simulink model "btp_VERSION2_final"  (R2020a)
settings: Solver=VariableStepAuto  StartTime=0.0  StopTime=14000  RelTol=1e-3
PreLoadFcn:
  | building_length = 15; % m
  | building_width = 10; % m
  | building_height = 2.5; % m
  | 
  | wall_thickness = 0.2; % m
  | wall_density = 2000; % kg/m^3
  | wall_specific_heat = 840; % J/(kg*K)
  | wall_conductivity = 0.04; % W/(m*K)
  | wall_heat_transfer_coeff_internal = 25; % W/(m^2*K)
  | wall_heat_transfer_coeff_external = 35; % W/(m^2*K)
  | 
  | roof_thickness = 0.2; % m
  | roof_density = 2000; % kg/m^3
  | roof_specific_heat = 840; % J/(kg*K)
  | roof_conductivity = 0.035; % W/(m*K)
  | roof_heat_transfer_coeff_internal = 10; % W/(m^2*K)
  | roof_heat_transfer_coeff_external = 30; % W/(m^2*K)
  | 
  | floor_thickness = 0.1; % m
  | floor_conductivity = 0.15; % W/(m*K)
  | floor_heat_transfer_coeff_internal = 15; % W/(m^2*K)
  | 
  | door_area = 2*0.6; % m^2
  | 
  | duct_area = 0.1^2; % m^2
  | 
  | fan_setting_table = 0 : 4; % 1
  | fan_flow_rate_table = [0 0.08 0.12 0.16 0.2]; % kg/s
  | 
  | initial_temperature = 35; % degC
  | ground_temperature = 25; % degC
  | 
  | flow_reversal_Mach = 1e-5; % 1
InitFcn:
  | zone_volume = building_length * building_width * building_height / 4; % m^3
  | zone_flow_area = 0.7 * building_height * (building_length + building_width) / 4; % m^2
model workspace (MAT data in the model file):
  building_height = 3
  building_length = 4.4
  building_width = 4
  door_area : Simulink.Parameter (value not decoded)
  duct_area = 0.02
  fan_flow_rate_table = [0 0.08 0.12 0.16 0.2]
  fan_setting_table = [0 1 2 3 4]
  floor_conductivity = 0.15
  floor_heat_transfer_coeff_internal = 15
  floor_thickness = 0.1
  flow_reversal_Mach = 1e-05
  ground_temperature = 27
  initial_temperature = 35
  roof_conductivity = 0.04
  roof_density = 2000
  roof_heat_transfer_coeff_external = 30
  roof_heat_transfer_coeff_internal = 10
  roof_specific_heat = 840
  roof_thickness = 0.2
  simlog_ssc_building_ventilation : simscape.logging.Node (value not decoded)
  tout = [0 3.15544362088e-30 8.45959628835e-09 2.5378788865e-08 3.73619145974e-08 4.93450403297e-08 6.73197289282e-08 8.52944175267e-08 1.12256450424e-07 1.39218483322e-07 1.6618051622e-07 1.93142549118e-07 ... (463 elements, 463x1)]
  wall_conductivity = 0.04
  wall_density = 2000
  wall_heat_transfer_coeff_external = 35
  wall_heat_transfer_coeff_internal = 25
  wall_specific_heat = 840
  wall_thickness = 0.2
  zone_flow_area = 9
  zone_volume = 50
undefined symbols (not defined in the file): dbresponses22S1, sigbuilder_block
libraries: fl_lib x53, nesl_utility x27, HVAC_lib x2, simulink x2, fuzblock x1
(part 2 of 2)

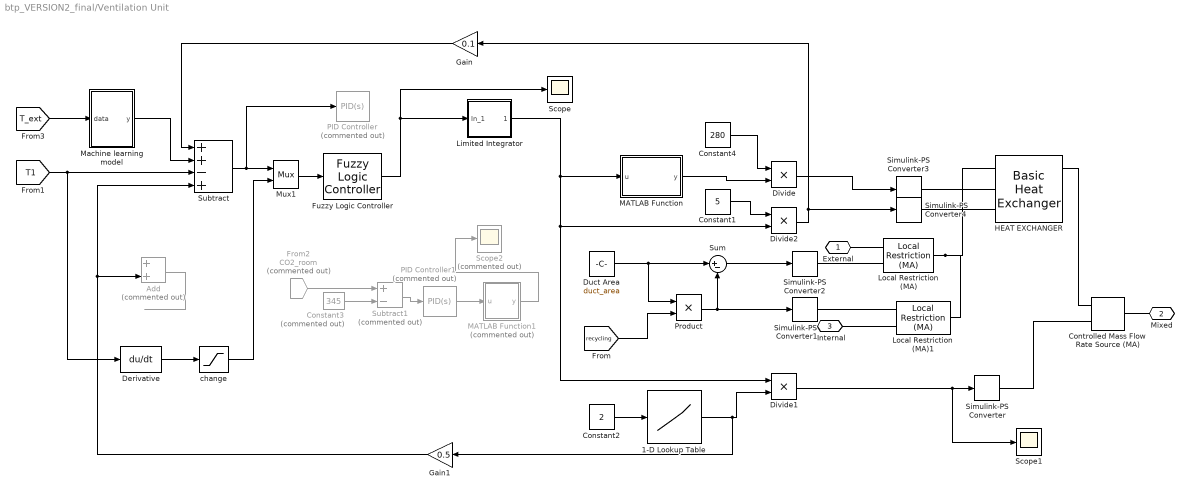
== system btp_VERSION2_final/Ventilation Unit ==
  1-D Lookup Table : Lookup_n-D  NumberOfTableDimensions=1  BreakpointsForDimension1=fan_setting_table  Table=fan_flow_rate_table  ExtrapMethod=Clip  InternalRulePriority=Speed  RndMeth=Simplest  InputSameDT=on
  Add : Sum  Commented=on
  Constant1 : Constant  Value=5
  Constant2 : Constant  Value=2
  Constant3 : Constant  Commented=on  Value=345
  Constant4 : Constant  Value=280
  Controlled Mass Flow Rate Source (MA) : fl_lib/Moist Air/Sources/Controlled Mass Flow Rate Source (MA)  power_spec=foundation.enum.power_spec.isentropic  area_A=duct_area m^2  area_B=duct_area m^2
      settings: SourceProductBaseCode=SS  InternalSimscapePortConfiguration="{\"Bottom\":[],\"Left\":[{\"id\":\"A\",\"label\":\"A\",\"type\":\"foundation.moist_air.moist_air\"},{\"id\":\"M\",\"label\":\"M\",\"type\":\"input\"}],\"Right\":[{\"id\":\"B\",\"label\":\"B\",\"type\":\"foundation.moist_air.moist_air\"}],\"Top\":[]}"
  Derivative : Derivative
  Divide : Product  Inputs=**
  Divide1 : Product  Inputs=**
  Divide2 : Product  Inputs=**
  Duct Area : Constant  Value=duct_area
  From2 : From  Commented=on  GotoTag=CO2_room  TagVisibility=global
  Fuzzy Logic Controller : fuzblock/Fuzzy Logic  Controller  FIS='tipper.fis'  OutputSampleNumber=101  DataType=double  FuzzifiedInputs=off  RuleFiringStrengths=off  RuleOutputs=off  AggregatedOutputs=off  SimulateUsing=Interpreted execution  OutOfRangeInputValueMessage=warning  NoRuleFiredMessage=warning  EmptyOutputFuzzySetMessage=warning
  Gain : Gain  Gain=0.1
  Gain1 : Gain  Gain=0.5
  HEAT EXCHANGER : HVAC_lib/Basic Heat Exchanger  Q_des=6 kW  T1_des=35 degC  mdot1_des=4 kg/s  cp1_des=2 kJ/kg/K  Dp1_des=0.8 kPa  T2_des=300 K  mdot2_des=20 kg/s  cp2_des=10 kJ/kg/K  volume=1e2 m^3  port_area=duct_area m^2  RH_ws=1  time_constant=1e-3 s  p_I_specify=off  p_I_priority=High  p_I=p_env atm  p_I_nominal_specify=off  p_I_nominal_unit=MPa  p_I_nominal_value=1  T_I_specify=on  T_I_priority=High  T_I=initial_temperature degC  T_I_nominal_specify=off  T_I_nominal_unit=K  T_I_nominal_value=1  RH_I_specify=on  RH_I_priority=High  RH_I=0.57  RH_I_nominal_specify=off  RH_I_nominal_unit=1  RH_I_nominal_value=1  x_w_I_specify=off  x_w_I_priority=None  x_w_I=0  x_w_I_nominal_specify=off  x_w_I_nominal_unit=1  x_w_I_nominal_value=1  y_w_I_specify=off  y_w_I_priority=None  y_w_I=0  y_w_I_nominal_specify=off  y_w_I_nominal_unit=1  y_w_I_nominal_value=1  HR_I_specify=off  HR_I_priority=None  HR_I=0  HR_I_nominal_specify=off  HR_I_nominal_unit=1  HR_I_nominal_value=1  x_g_I_specify=off  x_g_I_priority=None  x_g_I=0  x_g_I_nominal_specify=off  x_g_I_nominal_unit=1  x_g_I_nominal_value=1  y_g_I_specify=on  y_g_I_priority=None  y_g_I=0.00045  y_g_I_nominal_specify=off  y_g_I_nominal_unit=1  y_g_I_nominal_value=1
      settings: SourceProductBaseCode=SS  InternalSimscapePortConfiguration="{\"Bottom\":[],\"Left\":[{\"id\":\"A\",\"label\":\"A\",\"type\":\"foundation.moist_air.moist_air\"},{\"id\":\"T2\",\"label\":\"T2\",\"type\":\"input\"},{\"id\":\"M2\",\"label\":\"M2\",\"type\":\"input\"}],\"Right\":[{\"id\":\"B\",\"label\":\"B\",\"type\":\"foundation.moist_air.moist_air\"},{\"id\":\"W\",\"label\":\"W\",\"type\":\"output\"},{\"id\":\"F\",\"label\":\"F\",\"type\":\"output\"}],\"Top\":[]}"
  Limited Integrator : Subsystem  mask(Limited integrator.){lb=0.45, ub=2.95, xi=1}
      mask prompts: lb "Lower bound:"; ub "Upper bound:"; xi "Initial condition"
      mask help: Limited integrator
      mask Help: Implements a limited integrator with \nan expression of the form:\n\nif(x<=lb and u<0) or (x>=ub and u>0)\n\txdot=0\nelse\n\txdot=u.
      mask Display: plot(-1,-0.2,3.5,1.2,[0.05,1,2,2.9],[0,0,1,1]);disp(' 1/s    ')
  Local Restriction (MA) : fl_lib/Moist Air/Elements/Local Restriction (MA)  restriction_type=foundation.enum.restriction_type.variable  restriction_area=0.001 m^2  min_area=1e-10 m^2  max_area=0.99*duct_area m^2  area=duct_area m^2  Cd=0.8  B_lam=0.999
      settings: SourceProductBaseCode=SS
  Local Restriction (MA)1 : fl_lib/Moist Air/Elements/Local Restriction (MA)  restriction_type=foundation.enum.restriction_type.variable  restriction_area=0.001 m^2  min_area=1e-10 m^2  max_area=0.99 * duct_area m^2  area=duct_area m^2  Cd=0.8  B_lam=0.999
      settings: SourceProductBaseCode=SS
  MATLAB Function : MATLAB Function  TreatAsAtomicUnit=on
  MATLAB Function1 : MATLAB Function  Commented=on  TreatAsAtomicUnit=on
  Machine learning model : Subsystem
  Mux1 : Mux  Inputs=2
  PID Controller : simulink/Continuous/PID Controller  Commented=on  Controller=PID  Form=Parallel  TimeDomain=Continuous-time  UseExternalTs=off  SampleTime=-1  IntegratorMethod=Forward Euler  FilterMethod=Forward Euler  ControllerParametersSource=internal  P=4.6  I=0  D=0  UseFilter=on  N=100  TunerSelectOption=Transfer Function Based (PID Tuner App)  InitialConditionSource=internal  InitialConditionForIntegrator=0  InitialConditionForFilter=0  DifferentiatorICPrevScaledInput=0  ExternalReset=none  TrackingMode=off  Kt=1  LimitOutput=on  UpperSaturationLimit=1.25  LowerSaturationLimit=0.75  LinearizeAsGain=on  AntiWindupMode=none  Kb=1  POutMin=[]  POutMax=[]  IOutMin=[]  IOutMax=[]  DOutMin=[]  DOutMax=[]  NOutMin=[]  NOutMax=[]  SumOutMin=[]  SumOutMax=[]  SaturationOutMin=[]  SaturationOutMax=[]  PParamMin=[]  PParamMax=[]  IParamMin=[]  IParamMax=[]  DParamMin=[]  DParamMax=[]  NParamMin=[]  NParamMax=[]  KbParamMin=[]  KbParamMax=[]  KtParamMin=[]  KtParamMax=[]  KbOutMin=[]  KbOutMax=[]  KtOutMin=[]  KtOutMax=[]  IntegratorOutMin=[]  IntegratorOutMax=[]  FilterOutMin=[]  FilterOutMax=[]  SumI1OutMin=[]  SumI1OutMax=[]  SumI2OutMin=[]  SumI2OutMax=[]  SumI3OutMin=[]  SumI3OutMax=[]  SumI4OutMin=[]  SumI4OutMax=[]  SumDOutMin=[]  SumDOutMax=[]  DifferentiatorOutMin=[]  DifferentiatorOutMax=[]  FilterDiffOutCoefMin=[]  FilterDiffOutCoefMax=[]  ReciprocalOutMin=[]  ReciprocalOutMax=[]  SumDenOutMin=[]  SumDenOutMax=[]  SumNumOutMin=[]  SumNumOutMax=[]  DivideOutMin=[]  DivideOutMax=[]  UdiffTsProdOutMin=[]  UdiffTsProdOutMax=[]  NTsProdOutMin=[]  NTsProdOutMax=[]  UintegralTsProdOutMin=[]  UintegralTsProdOutMax=[]  UngainTsProdOutMin=[]  UngainTsProdOutMax=[]  IntegratorContinuousStateAttributes=''  IntegratorStateMustResolveToSignalObject=off  IntegratorRTWStateStorageClass=Auto  FilterContinuousStateAttributes=''  FilterStateMustResolveToSignalObject=off  FilterRTWStateStorageClass=Auto  ParallelPVariant=InternalParameters  IdealPVariant=Disabled  IVariant=InternalParameters  DVariant=InternalParameters  IntegratorVariant=Continuous  SatVariant=Enabled  AWVariant=Passthrough  PCopyVariant=Disabled  TRVariant=Disabled  FdbkBlocksVariant=Forward  IdealPFdbkVariant=Disabled  SatFdbkVariant=Disabled  DerivativeFilterVariant=ContFilter  NVariant=InternalParameters  NCopyVariant=Disabled  FilterICVariant=InternalICsFilter  IntegratorICVariant=InternalICs  ExternalResetVariant=Disabled  TRSumVariant=Passthrough  SumFdbkVariant=Disabled  SumVariant=Sum_PID  TsampFilterVariant=InternalTs  TsampNgainVariant=Passthrough  TsampIntegralVariant=Passthrough
  PID Controller1 : simulink/Continuous/PID Controller  Commented=on  Controller=PID  Form=Parallel  TimeDomain=Continuous-time  UseExternalTs=off  SampleTime=-1  IntegratorMethod=Forward Euler  FilterMethod=Forward Euler  ControllerParametersSource=internal  P=5  I=0.02  D=0  UseFilter=on  N=100  TunerSelectOption=Transfer Function Based (PID Tuner App)  InitialConditionSource=internal  InitialConditionForIntegrator=0  InitialConditionForFilter=0  DifferentiatorICPrevScaledInput=0  ExternalReset=none  TrackingMode=off  Kt=1  LimitOutput=on  UpperSaturationLimit=1.20  LowerSaturationLimit=0.8  LinearizeAsGain=on  AntiWindupMode=none  Kb=1  POutMin=[]  POutMax=[]  IOutMin=[]  IOutMax=[]  DOutMin=[]  DOutMax=[]  NOutMin=[]  NOutMax=[]  SumOutMin=[]  SumOutMax=[]  SaturationOutMin=[]  SaturationOutMax=[]  PParamMin=[]  PParamMax=[]  IParamMin=[]  IParamMax=[]  DParamMin=[]  DParamMax=[]  NParamMin=[]  NParamMax=[]  KbParamMin=[]  KbParamMax=[]  KtParamMin=[]  KtParamMax=[]  KbOutMin=[]  KbOutMax=[]  KtOutMin=[]  KtOutMax=[]  IntegratorOutMin=[]  IntegratorOutMax=[]  FilterOutMin=[]  FilterOutMax=[]  SumI1OutMin=[]  SumI1OutMax=[]  SumI2OutMin=[]  SumI2OutMax=[]  SumI3OutMin=[]  SumI3OutMax=[]  SumI4OutMin=[]  SumI4OutMax=[]  SumDOutMin=[]  SumDOutMax=[]  DifferentiatorOutMin=[]  DifferentiatorOutMax=[]  FilterDiffOutCoefMin=[]  FilterDiffOutCoefMax=[]  ReciprocalOutMin=[]  ReciprocalOutMax=[]  SumDenOutMin=[]  SumDenOutMax=[]  SumNumOutMin=[]  SumNumOutMax=[]  DivideOutMin=[]  DivideOutMax=[]  UdiffTsProdOutMin=[]  UdiffTsProdOutMax=[]  NTsProdOutMin=[]  NTsProdOutMax=[]  UintegralTsProdOutMin=[]  UintegralTsProdOutMax=[]  UngainTsProdOutMin=[]  UngainTsProdOutMax=[]  IntegratorContinuousStateAttributes=''  IntegratorStateMustResolveToSignalObject=off  IntegratorRTWStateStorageClass=Auto  FilterContinuousStateAttributes=''  FilterStateMustResolveToSignalObject=off  FilterRTWStateStorageClass=Auto  ParallelPVariant=InternalParameters  IdealPVariant=Disabled  IVariant=InternalParameters  DVariant=InternalParameters  IntegratorVariant=Continuous  SatVariant=Enabled  AWVariant=Passthrough  PCopyVariant=Disabled  TRVariant=Disabled  FdbkBlocksVariant=Forward  IdealPFdbkVariant=Disabled  SatFdbkVariant=Disabled  DerivativeFilterVariant=ContFilter  NVariant=InternalParameters  NCopyVariant=Disabled  FilterICVariant=InternalICsFilter  IntegratorICVariant=InternalICs  ExternalResetVariant=Disabled  TRSumVariant=Passthrough  SumFdbkVariant=Disabled  SumVariant=Sum_PID  TsampFilterVariant=InternalTs  TsampNgainVariant=Passthrough  TsampIntegralVariant=Passthrough
  Product : Product
  Scope : Scope
  Scope1 : Scope
  Scope2 : Scope  Commented=on
  Simulink-PS Converter : nesl_utility/Simulink-PS Converter  PhysicalDomain=network_engine_domain  SubClassName=ps_input  LeftPortType=input  RightPortType=output  PseudoPeriodic=off  Frequencies=[]  NoiseDistribution=none  NoiseParameters=[]  Unit=kg/s  AffineConversion=off  FilteringAndDerivatives=provide  SimscapeFilterOrder=1  InputFilterTimeConstant=0.001  UdotUserProvided=0
  Simulink-PS Converter1 : nesl_utility/Simulink-PS Converter  PhysicalDomain=network_engine_domain  SubClassName=ps_input  LeftPortType=input  RightPortType=output  PseudoPeriodic=off  Frequencies=[]  NoiseDistribution=none  NoiseParameters=[]  Unit=m^2  AffineConversion=off  FilteringAndDerivatives=provide  SimscapeFilterOrder=1  InputFilterTimeConstant=0.001  UdotUserProvided=0
  Simulink-PS Converter2 : nesl_utility/Simulink-PS Converter  PhysicalDomain=network_engine_domain  SubClassName=ps_input  LeftPortType=input  RightPortType=output  PseudoPeriodic=off  Frequencies=[]  NoiseDistribution=none  NoiseParameters=[]  Unit=m^2  AffineConversion=off  FilteringAndDerivatives=provide  SimscapeFilterOrder=1  InputFilterTimeConstant=0.001  UdotUserProvided=0
  Simulink-PS Converter3 : nesl_utility/Simulink-PS Converter  PhysicalDomain=network_engine_domain  SubClassName=ps_input  LeftPortType=input  RightPortType=output  PseudoPeriodic=off  Frequencies=[]  NoiseDistribution=none  NoiseParameters=[]  Unit=K  AffineConversion=on  FilteringAndDerivatives=provide  SimscapeFilterOrder=1  InputFilterTimeConstant=0.001  UdotUserProvided=0
  Simulink-PS Converter4 : nesl_utility/Simulink-PS Converter  PhysicalDomain=network_engine_domain  SubClassName=ps_input  LeftPortType=input  RightPortType=output  PseudoPeriodic=off  Frequencies=[]  NoiseDistribution=none  NoiseParameters=[]  Unit=kg/s  AffineConversion=on  FilteringAndDerivatives=provide  SimscapeFilterOrder=1  InputFilterTimeConstant=0.001  UdotUserProvided=0
  Subtract : Sum  Inputs=++-+
  Subtract1 : Sum  Commented=on  Inputs=+-
  Sum : Sum  Inputs=|+-
  change : Saturate  UpperLimit=2  LowerLimit=-2
  External : PMIOPort  Side=Left
  Mixed : PMIOPort  Port=2  Side=Right
  Internal : PMIOPort  Port=3  Side=Left
  wires:
  Product/1 -> Sum/2, Simulink-PS Converter1/1
  Sum/1 -> Simulink-PS Converter2/1
  Duct Area/1 -> Product/1, Sum/1
  Constant4/1 -> Divide/1
  [T1] -> Derivative/1, Subtract/3
  Subtract/1 -> PID Controller/1, Mux1/1
  Divide2/1 -> Gain/1, Simulink-PS Converter4/1
  Divide/1 -> Simulink-PS Converter3/1
  Divide1/1 -> Simulink-PS Converter/1, Scope1/1
  Constant2/1 -> 1-D Lookup Table/1
  Constant3/1 -> Subtract1/2
  From2/1 -> Subtract1/1
  Subtract1/1 -> PID Controller1/1
  PID Controller1/1 -> MATLAB Function1/1(u)
  MATLAB Function1/1(y) -> Scope2/1
  [recycling] -> Product/2
  Gain/1 -> Subtract/1
  1-D Lookup Table/1 -> Gain1/1, Divide1/2
  Gain1/1 -> Add/2, Subtract/4
  Derivative/1 -> change/1
  change/1 -> Mux1/2
  Mux1/1 -> Fuzzy Logic Controller/1
  Fuzzy Logic Controller/1 -> Limited Integrator/1(In_1), Scope/1
  Limited Integrator/1(Out_1) -> MATLAB Function/1(u), Divide2/2, Divide1/1
  Constant1/1 -> Divide2/1
  Machine learning model/1(y) -> Subtract/2
  [T_ext] -> Machine learning model/1(data)
  MATLAB Function/1(y) -> Divide/2
  Add/1 -> ?
  connections:
  Simulink-PS Converter/RConn1 -- Controlled Mass Flow Rate Source (MA)/LConn2
  External/RConn1 -- Local Restriction (MA)/LConn1
  Simulink-PS Converter2/RConn1 -- Local Restriction (MA)/LConn2
  Controlled Mass Flow Rate Source (MA)/RConn1 -- Mixed/RConn1
  Simulink-PS Converter1/RConn1 -- Local Restriction (MA)1/LConn2
  Internal/RConn1 -- Local Restriction (MA)1/LConn1
  Local Restriction (MA)/RConn1 -- HEAT EXCHANGER/LConn1 -- Local Restriction (MA)1/RConn1
  Simulink-PS Converter3/RConn1 -- HEAT EXCHANGER/LConn2
  Simulink-PS Converter4/RConn1 -- HEAT EXCHANGER/LConn3
  HEAT EXCHANGER/RConn1 -- Controlled Mass Flow Rate Source (MA)/LConn1

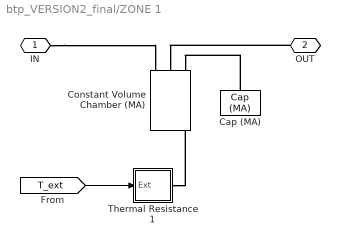
== system btp_VERSION2_final/ZONE 1 ==
  Cap (MA) : fl_lib/Moist Air/Elements/Cap (MA)  p_specify=on  p_priority=None  p=0.101325 MPa  p_nominal_specify=off  p_nominal_unit=MPa  p_nominal_value=1  T_specify=on  T_priority=None  T=initial_temperature K  T_nominal_specify=off  T_nominal_unit=K  T_nominal_value=1  x_w_specify=on  x_w_priority=None  x_w=0.57  x_w_nominal_specify=off  x_w_nominal_unit=1  x_w_nominal_value=1  x_g_specify=on  x_g_priority=None  x_g=0.00045  x_g_nominal_specify=off  x_g_nominal_unit=1  x_g_nominal_value=1
      settings: SourceProductBaseCode=SS  InternalSimscapePortConfiguration="{\"Bottom\":[],\"Left\":[{\"id\":\"A\",\"label\":\"\",\"type\":\"foundation.moist_air.moist_air\"}],\"Right\":[],\"Top\":[]}"
  Constant Volume Chamber (MA) : fl_lib/Moist Air/Elements/Constant Volume Chamber (MA)  volume=zone_volume/2 m^3  num_ports=foundation.enum.num_ports.three  area_A=duct_area m^2  area_B=zone_flow_area m^2  area_C=zone_flow_area m^2  area_D=0.01 m^2  RH_ws=1  time_constant=1e-3 s  moisture_trace_gas_source=foundation.enum.moisture_trace_gas_source.none  moisture_source_spec=foundation.enum.moisture_source_spec.vapor  moisture_mass_flow=0 kg/s  moisture_temperature_spec=foundation.enum.temperature_spec.atmospheric  moisture_temperature=293.15 K  trace_gas_mass_flow=0 kg/s  trace_gas_temperature_spec=foundation.enum.temperature_spec.atmospheric  trace_gas_temperature=293.15 K  p_I_specify=on  p_I_priority=High  p_I=0.101325 MPa  p_I_nominal_specify=off  p_I_nominal_unit=MPa  p_I_nominal_value=1  T_I_specify=on  T_I_priority=None  T_I=initial_temperature K  T_I_nominal_specify=off  T_I_nominal_unit=K  T_I_nominal_value=1  RH_I_specify=on  RH_I_priority=None  RH_I=0.57  RH_I_nominal_specify=off  RH_I_nominal_unit=1  RH_I_nominal_value=1  x_w_I_specify=off  x_w_I_priority=None  x_w_I=0  x_w_I_nominal_specify=off  x_w_I_nominal_unit=1  x_w_I_nominal_value=1  y_w_I_specify=off  y_w_I_priority=None  y_w_I=0  y_w_I_nominal_specify=off  y_w_I_nominal_unit=1  y_w_I_nominal_value=1  HR_I_specify=off  HR_I_priority=None  HR_I=0  HR_I_nominal_specify=off  HR_I_nominal_unit=1  HR_I_nominal_value=1  x_g_I_specify=off  x_g_I_priority=Low  x_g_I=0  x_g_I_nominal_specify=off  x_g_I_nominal_unit=1  x_g_I_nominal_value=1  y_g_I_specify=on  y_g_I_priority=None  y_g_I=0.00045  y_g_I_nominal_specify=off  y_g_I_nominal_unit=1  y_g_I_nominal_value=1
      settings: SourceProductBaseCode=SS  InternalSimscapePortConfiguration="{\"Bottom\":[],\"Left\":[{\"id\":\"A\",\"label\":\"A\",\"type\":\"foundation.moist_air.moist_air\"},{\"id\":\"B\",\"label\":\"B\",\"type\":\"foundation.moist_air.moist_air\"},{\"id\":\"C\",\"label\":\"C\",\"type\":\"foundation.moist_air.moist_air\"}],\"Right\":[{\"id\":\"W\",\"label\":\"W\",\"type\":\"output\"},{\"id\":\"F\",\"label\":\"F\",\"type\":\"output\"},{\"id\":\"H\",\"label\":\"H\",\"type\":\"foundation.thermal.thermal\"}],\"Top\":[]}"
  Thermal Resistance 1 : Subsystem  Tag=PublishSubsystem  mask(Zone Thermal Resistance){zone_length=building_length / 2, zone_width=building_width / 2, zone_height=building_height / 2, wall_thickness=wall_thickness, wall_density=wall_density, wall_specific_heat=wall_specific_heat, wall_conductivity=wall_conductivity, wall_heat_transfer_coeff_internal=wall_heat_transfer_coeff_internal, wall_heat_transfer_coeff_external=wall_heat_transfer_coeff_external, wall_initial_temperature=initial_temperature, roof_thickness=roof_thickness, roof_density=roof_density, roof_specific_heat=roof_specific_heat, roof_conductivity=roof_conductivity, roof_heat_transfer_coeff_internal=roof_heat_transfer_coeff_internal, roof_heat_transfer_coeff_external=roof_heat_transfer_coeff_external, roof_initial_temperature=initial_temperature, floor_thickness=floor_thickness, floor_conductivity=floor_conductivity, floor_heat_transfer_coeff_internal=floor_heat_transfer_coeff_internal, ground_temperature=ground_temperature}
      mask prompts: zone_length "Zone length (m)"; zone_width "Zone width (m)"; zone_height "Zone height (m)"; wall_thickness "Thickness (m)"; wall_density "Density (kg/m^3)"; wall_specific_heat "Specific heat (J/(kg*K))"; wall_conductivity "Thermal conductivity (W/(m*K))"; wall_heat_transfer_coeff_internal "Internal heat transfer coefficient (W/(m^2*K))"; wall_heat_transfer_coeff_external "External heat transfer coefficient (W/(m^2*K))"; wall_initial_temperature "Initial temperature (degC)"; roof_thickness "Thickness (m)"; roof_density "Density (kg/m^3)"; roof_specific_heat "Specific heat (J/(kg*K))"; roof_conductivity "Thermal conductivity (W/(m*K))"; roof_heat_transfer_coeff_internal "Internal heat transfer coefficient (W/(m^2*K))"; roof_heat_transfer_coeff_external "External heat transfer coefficient (W/(m^2*K))"; roof_initial_temperature "Initial temperature (degC)"; floor_thickness "Thickness (m)"; floor_conductivity "Thermal conductivity (W/(m*K))"; floor_heat_transfer_coeff_internal "Internal heat transfer coefficient (W/(m^2*K))"; ground_temperature "Ground temperature (degC)"
      mask help: This subsystem models the thermal resistances of the wall and of the roof between the zone and the external environment. It also models the thermal resistance of the floor between the zone and the ground.
      mask init:
      | wall_area = zone_height * (zone_length + zone_width);
      | roof_area = zone_length * zone_width;
      | floor_area = zone_length * zone_width;
      mask DialogControl TabGeometry Prompt: Geometry
      mask DialogControl TabWall Prompt: Wall
      mask DialogControl TabRoof Prompt: Roof
      mask DialogControl TabFloor Prompt: Floor
  IN : PMIOPort  Side=Left
  OUT : PMIOPort  Port=2  Side=Right
  wires:
  [T_ext] -> Thermal Resistance 1/1(Ext)
  connections:
  OUT/RConn1 -- Constant Volume Chamber (MA)/LConn2
  Cap (MA)/LConn1 -- Constant Volume Chamber (MA)/LConn3
  Thermal Resistance 1/RConn1 -- Constant Volume Chamber (MA)/RConn3
  IN/RConn1 -- Constant Volume Chamber (MA)/LConn1

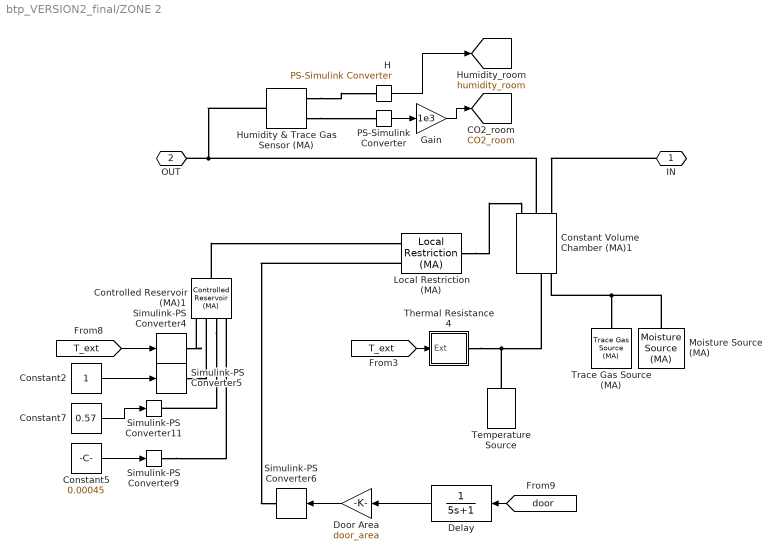
== system btp_VERSION2_final/ZONE 2 ==
  Constant Volume Chamber (MA)1 : fl_lib/Moist Air/Elements/Constant Volume Chamber (MA)  volume=zone_volume/2 m^3  num_ports=foundation.enum.num_ports.three  area_A=duct_area m^2  area_B=zone_flow_area m^2  area_C=zone_flow_area m^2  area_D=0.01 m^2  RH_ws=1  time_constant=1e-3 s  moisture_trace_gas_source=foundation.enum.moisture_trace_gas_source.controlled  moisture_source_spec=foundation.enum.moisture_source_spec.vapor  moisture_mass_flow=0 kg/s  moisture_temperature_spec=foundation.enum.temperature_spec.atmospheric  moisture_temperature=293.15 K  trace_gas_mass_flow=0 kg/s  trace_gas_temperature_spec=foundation.enum.temperature_spec.atmospheric  trace_gas_temperature=293.15 K  p_I_specify=on  p_I_priority=High  p_I=0.101325 MPa  p_I_nominal_specify=off  p_I_nominal_unit=MPa  p_I_nominal_value=1  T_I_specify=on  T_I_priority=High  T_I=initial_temperature K  T_I_nominal_specify=off  T_I_nominal_unit=K  T_I_nominal_value=1  RH_I_specify=on  RH_I_priority=None  RH_I=0.57  RH_I_nominal_specify=off  RH_I_nominal_unit=1  RH_I_nominal_value=1  x_w_I_specify=off  x_w_I_priority=None  x_w_I=0  x_w_I_nominal_specify=off  x_w_I_nominal_unit=1  x_w_I_nominal_value=1  y_w_I_specify=off  y_w_I_priority=None  y_w_I=0  y_w_I_nominal_specify=off  y_w_I_nominal_unit=1  y_w_I_nominal_value=1  HR_I_specify=off  HR_I_priority=None  HR_I=0  HR_I_nominal_specify=off  HR_I_nominal_unit=1  HR_I_nominal_value=1  x_g_I_specify=off  x_g_I_priority=None  x_g_I=0  x_g_I_nominal_specify=off  x_g_I_nominal_unit=1  x_g_I_nominal_value=1  y_g_I_specify=on  y_g_I_priority=None  y_g_I=0.00045  y_g_I_nominal_specify=off  y_g_I_nominal_unit=1  y_g_I_nominal_value=1
      settings: SourceProductBaseCode=SS  InternalSimscapePortConfiguration="{\"Bottom\":[],\"Left\":[{\"id\":\"A\",\"label\":\"A\",\"type\":\"foundation.moist_air.moist_air\"},{\"id\":\"B\",\"label\":\"B\",\"type\":\"foundation.moist_air.moist_air\"},{\"id\":\"C\",\"label\":\"C\",\"type\":\"foundation.moist_air.moist_air\"}],\"Right\":[{\"id\":\"W\",\"label\":\"W\",\"type\":\"output\"},{\"id\":\"F\",\"label\":\"F\",\"type\":\"output\"},{\"id\":\"H\",\"label\":\"H\",\"type\":\"foundation.thermal.thermal\"},{\"id\":\"S\",\"label\":\"S\",\"type\":\"foundation.moist_air.moist_air_source\"}],\"Top\":[]}"
  Constant2 : Constant
  Constant5 : Constant  Value=0.00045
  Constant7 : Constant  Value=0.57
  Controlled Reservoir (MA)1 : fl_lib/Moist Air/Elements/Controlled Reservoir (MA)  moisture_spec=foundation.enum.moisture_spec.relative_humidity  trace_gas_spec=foundation.enum.trace_gas_spec.mole_fraction  RH_ws=1  area_A=duct_area m^2  input_error_spec=foundation.enum.input_range_error.warn
      settings: SourceProductBaseCode=SS  InternalSimscapePortConfiguration="{\"Bottom\":[],\"Left\":[{\"id\":\"A\",\"label\":\"A\",\"type\":\"foundation.moist_air.moist_air\"}],\"Right\":[{\"id\":\"T\",\"label\":\"T\",\"type\":\"input\"},{\"id\":\"P\",\"label\":\"P\",\"type\":\"input\"},{\"id\":\"W\",\"label\":\"W\",\"type\":\"input\"},{\"id\":\"G\",\"label\":\"G\",\"type\":\"input\"}],\"Top\":[]}"
  Delay : TransferFcn  Denominator=[5 1]
  Door Area : Gain  Gain=door_area
  Gain : Gain  Gain=1e3
  H : nesl_utility/PS-Simulink Converter  PhysicalDomain=network_engine_domain  SubClassName=ps_output  LeftPortType=input  RightPortType=output  PseudoPeriodic=off  Frequencies=[]  Unit=1  AffineConversion=off
  Humidity & Trace Gas Sensor (MA) : fl_lib/Moist Air/Sensors/Humidity & Trace Gas Sensor (MA)  moisture_spec=foundation.enum.moisture_spec.relative_humidity  trace_gas_spec=foundation.enum.trace_gas_spec.mole_fraction
      settings: SourceProductBaseCode=SS  InternalSimscapePortConfiguration="{\"Bottom\":[],\"Left\":[{\"id\":\"A\",\"label\":\"A\",\"type\":\"foundation.moist_air.moist_air\"}],\"Right\":[{\"id\":\"W\",\"label\":\"W\",\"type\":\"output\"},{\"id\":\"G\",\"label\":\"G\",\"type\":\"output\"}],\"Top\":[]}"
  Local Restriction (MA) : fl_lib/Moist Air/Elements/Local Restriction (MA)  restriction_type=foundation.enum.restriction_type.variable  restriction_area=0.5 * duct_area m^2  min_area=1e-7 m^2  max_area=0.9*door_area m^2  area=door_area m^2  Cd=0.8  B_lam=0.999
      settings: SourceProductBaseCode=SS
  Moisture Source (MA) : fl_lib/Moist Air/Sources/Moisture & Trace Gas Sources/Moisture Source (MA)  moisture_source_spec=foundation.enum.moisture_source_spec.vapor  moisture_mass_flow=0.015 kg/s  temperature_spec=foundation.enum.temperature_spec.specified  moisture_temperature=303 K
      settings: SourceProductBaseCode=SS  InternalSimscapePortConfiguration="{\"Bottom\":[],\"Left\":[{\"id\":\"S\",\"label\":\"S\",\"type\":\"foundation.moist_air.moist_air_source\"}],\"Right\":[],\"Top\":[]}"
  PS-Simulink Converter : nesl_utility/PS-Simulink Converter  PhysicalDomain=network_engine_domain  SubClassName=ps_output  LeftPortType=input  RightPortType=output  PseudoPeriodic=off  Frequencies=[]  Unit=1  AffineConversion=off
  Simulink-PS Converter11 : nesl_utility/Simulink-PS Converter  PhysicalDomain=network_engine_domain  SubClassName=ps_input  LeftPortType=input  RightPortType=output  PseudoPeriodic=off  Frequencies=[]  NoiseDistribution=none  NoiseParameters=[]  Unit=1  AffineConversion=off  FilteringAndDerivatives=provide  SimscapeFilterOrder=1  InputFilterTimeConstant=0.001  UdotUserProvided=0
  Simulink-PS Converter4 : nesl_utility/Simulink-PS Converter  PhysicalDomain=network_engine_domain  SubClassName=ps_input  LeftPortType=input  RightPortType=output  PseudoPeriodic=off  Frequencies=[]  NoiseDistribution=none  NoiseParameters=[]  Unit=degC  AffineConversion=on  FilteringAndDerivatives=provide  SimscapeFilterOrder=1  InputFilterTimeConstant=0.001  UdotUserProvided=0
  Simulink-PS Converter5 : nesl_utility/Simulink-PS Converter  PhysicalDomain=network_engine_domain  SubClassName=ps_input  LeftPortType=input  RightPortType=output  PseudoPeriodic=off  Frequencies=[]  NoiseDistribution=none  NoiseParameters=[]  Unit=atm  AffineConversion=off  FilteringAndDerivatives=provide  SimscapeFilterOrder=1  InputFilterTimeConstant=0.001  UdotUserProvided=0
  Simulink-PS Converter6 : nesl_utility/Simulink-PS Converter  PhysicalDomain=network_engine_domain  SubClassName=ps_input  LeftPortType=input  RightPortType=output  PseudoPeriodic=off  Frequencies=[]  NoiseDistribution=none  NoiseParameters=[]  Unit=m^2  AffineConversion=off  FilteringAndDerivatives=provide  SimscapeFilterOrder=1  InputFilterTimeConstant=0.001  UdotUserProvided=0
  Simulink-PS Converter9 : nesl_utility/Simulink-PS Converter  PhysicalDomain=network_engine_domain  SubClassName=ps_input  LeftPortType=input  RightPortType=output  PseudoPeriodic=off  Frequencies=[]  NoiseDistribution=none  NoiseParameters=[]  Unit=1  AffineConversion=off  FilteringAndDerivatives=provide  SimscapeFilterOrder=1  InputFilterTimeConstant=0.001  UdotUserProvided=0
  Temperature Source : fl_lib/Thermal/Thermal Sources/Temperature Source  temperature=303 K
  Thermal Resistance 4 : Subsystem  mask(Zone Thermal Resistance){zone_length=building_length / 2, zone_width=building_width / 2, zone_height=building_height / 2, wall_thickness=wall_thickness, wall_density=wall_density, wall_specific_heat=wall_specific_heat, wall_conductivity=wall_conductivity, wall_heat_transfer_coeff_internal=wall_heat_transfer_coeff_internal, wall_heat_transfer_coeff_external=wall_heat_transfer_coeff_external, wall_initial_temperature=initial_temperature, roof_thickness=roof_thickness, roof_density=roof_density, roof_specific_heat=roof_specific_heat, roof_conductivity=roof_conductivity, roof_heat_transfer_coeff_internal=roof_heat_transfer_coeff_internal, roof_heat_transfer_coeff_external=roof_heat_transfer_coeff_external, roof_initial_temperature=initial_temperature, floor_thickness=floor_thickness, floor_conductivity=floor_conductivity, floor_heat_transfer_coeff_internal=floor_heat_transfer_coeff_internal, ground_temperature=ground_temperature}
      mask prompts: zone_length "Zone length (m)"; zone_width "Zone width (m)"; zone_height "Zone height (m)"; wall_thickness "Thickness (m)"; wall_density "Density (kg/m^3)"; wall_specific_heat "Specific heat (J/(kg*K))"; wall_conductivity "Thermal conductivity (W/(m*K))"; wall_heat_transfer_coeff_internal "Internal heat transfer coefficient (W/(m^2*K))"; wall_heat_transfer_coeff_external "External heat transfer coefficient (W/(m^2*K))"; wall_initial_temperature "Initial temperature (degC)"; roof_thickness "Thickness (m)"; roof_density "Density (kg/m^3)"; roof_specific_heat "Specific heat (J/(kg*K))"; roof_conductivity "Thermal conductivity (W/(m*K))"; roof_heat_transfer_coeff_internal "Internal heat transfer coefficient (W/(m^2*K))"; roof_heat_transfer_coeff_external "External heat transfer coefficient (W/(m^2*K))"; roof_initial_temperature "Initial temperature (degC)"; floor_thickness "Thickness (m)"; floor_conductivity "Thermal conductivity (W/(m*K))"; floor_heat_transfer_coeff_internal "Internal heat transfer coefficient (W/(m^2*K))"; ground_temperature "Ground temperature (degC)"
      mask help: This subsystem models the thermal resistances of the wall and of the roof between the zone and the external environment. It also models the thermal resistance of the floor between the zone and the ground.
      mask init:
      | wall_area = zone_height * (zone_length + zone_width);
      | roof_area = zone_length * zone_width;
      | floor_area = zone_length * zone_width;
      mask DialogControl TabGeometry Prompt: Geometry
      mask DialogControl TabWall Prompt: Wall
      mask DialogControl TabRoof Prompt: Roof
      mask DialogControl TabFloor Prompt: Floor
  Trace Gas Source (MA) : fl_lib/Moist Air/Sources/Moisture & Trace Gas Sources/Trace Gas Source (MA)  trace_gas_mass_flow=0.04 kg/s  temperature_spec=foundation.enum.temperature_spec.specified  trace_gas_temperature=303 K
      settings: SourceProductBaseCode=SS  InternalSimscapePortConfiguration="{\"Bottom\":[],\"Left\":[{\"id\":\"S\",\"label\":\"S\",\"type\":\"foundation.moist_air.moist_air_source\"}],\"Right\":[],\"Top\":[]}"
  IN : PMIOPort  Side=Right
  OUT : PMIOPort  Port=2  Side=Left
  tag scope: CO2_room=global, humidity_room=global
  wires:
  Constant2/1 -> Simulink-PS Converter5/1
  Delay/1 -> Door Area/1
  Constant5/1 -> Simulink-PS Converter9/1
  [T_ext] -> Thermal Resistance 4/1(Ext)
  Constant7/1 -> Simulink-PS Converter11/1
  PS-Simulink Converter/1 -> Gain/1
  H/1 -> [humidity_room]
  Door Area/1 -> Simulink-PS Converter6/1
  [T_ext] -> Simulink-PS Converter4/1
  [door] -> Delay/1
  Gain/1 -> [CO2_room]
  connections:
  Controlled Reservoir (MA)1/LConn1 -- Local Restriction (MA)/LConn1
  Humidity & Trace Gas Sensor (MA)/RConn1 -- H/LConn1
  Controlled Reservoir (MA)1/RConn3 -- Simulink-PS Converter11/RConn1
  Simulink-PS Converter9/RConn1 -- Controlled Reservoir (MA)1/RConn4
  Thermal Resistance 4/RConn1 -- Temperature Source/LConn1 -- Constant Volume Chamber (MA)1/RConn3
  Humidity & Trace Gas Sensor (MA)/LConn1 -- Constant Volume Chamber (MA)1/LConn2 -- OUT/RConn1
  Local Restriction (MA)/LConn2 -- Simulink-PS Converter6/RConn1
  Local Restriction (MA)/RConn1 -- Constant Volume Chamber (MA)1/LConn1
  Moisture Source (MA)/LConn1 -- Constant Volume Chamber (MA)1/RConn4 -- Trace Gas Source (MA)/LConn1
  Humidity & Trace Gas Sensor (MA)/RConn2 -- PS-Simulink Converter/LConn1
  Simulink-PS Converter5/RConn1 -- Controlled Reservoir (MA)1/RConn2
  Simulink-PS Converter4/RConn1 -- Controlled Reservoir (MA)1/RConn1
  IN/RConn1 -- Constant Volume Chamber (MA)1/LConn3

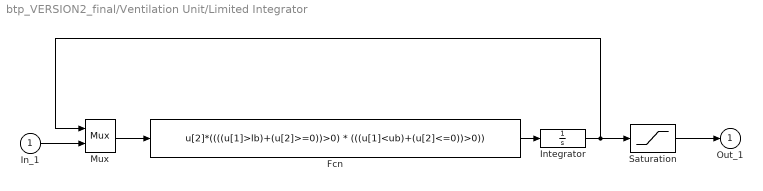
== system btp_VERSION2_final/Ventilation Unit/Limited Integrator ==
  In_1 : Inport
  Fcn : Fcn  Expr=u[2]*((((u[1]>lb)+(u[2]>=0))>0) * (((u[1]<ub)+(u[2]<=0))>0))
  Integrator : Integrator  InitialCondition=xi
  Mux : Mux  Inputs=2
  Saturation : Saturate  UpperLimit=ub  LowerLimit=lb
  Out_1 : Outport  InitialOutput=0  VectorParamsAs1DForOutWhenUnconnected=off
  wires:
  Integrator/1 -> Saturation/1, Mux/1
  Fcn/1 -> Integrator/1
  Mux/1 -> Fcn/1
  In_1/1 -> Mux/2
  Saturation/1 -> Out_1/1

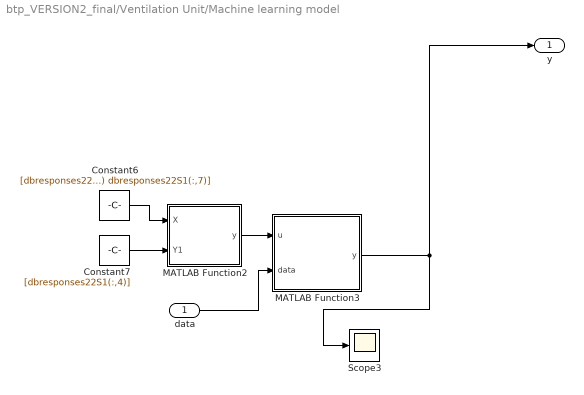
== system btp_VERSION2_final/Ventilation Unit/Machine learning model ==
  data : Inport
  Constant6 : Constant  Value=[dbresponses22S1(:,1) dbresponses22S1(:,2) dbresponses22S1(:,5) dbresponses22S1(:,6) dbresponses22S1(:,7)]
  Constant7 : Constant  Value=[dbresponses22S1(:,4)]
  MATLAB Function2 : MATLAB Function  TreatAsAtomicUnit=on
  MATLAB Function3 : MATLAB Function  TreatAsAtomicUnit=on
  Scope3 : Scope
  y : Outport
  wires:
  MATLAB Function3/1(y) -> y/1, Scope3/1
  MATLAB Function2/1(y) -> MATLAB Function3/1(u)
  Constant6/1 -> MATLAB Function2/1(X)
  data/1 -> MATLAB Function3/2(data)
  Constant7/1 -> MATLAB Function2/2(Y1)

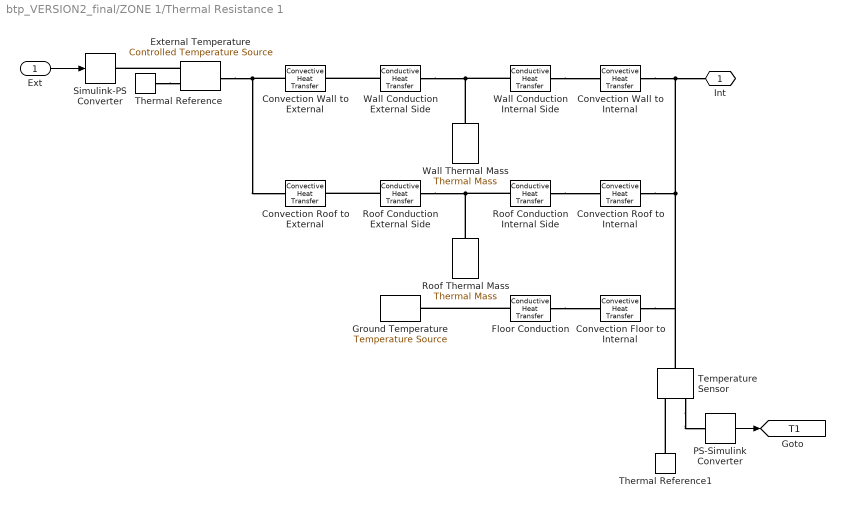
== system btp_VERSION2_final/ZONE 1/Thermal Resistance 1 ==
  Ext : Inport
  Convection Floor to Internal : fl_lib/Thermal/Thermal Elements/Convective Heat Transfer  area=floor_area m^2  heat_tr_coeff=floor_heat_transfer_coeff_internal W/(m^2 * K)  T_specify=off  T_priority=None  T=0 K  T_nominal_specify=off  T_nominal_unit=K  T_nominal_value=1  Q_specify=off  Q_priority=None  Q=0 W  Q_nominal_specify=off  Q_nominal_unit=W  Q_nominal_value=1
  Convection Roof to External : fl_lib/Thermal/Thermal Elements/Convective Heat Transfer  area=roof_area m^2  heat_tr_coeff=roof_heat_transfer_coeff_external W/(m^2 * K)  T_specify=off  T_priority=None  T=0 K  T_nominal_specify=off  T_nominal_unit=K  T_nominal_value=1  Q_specify=off  Q_priority=None  Q=0 W  Q_nominal_specify=off  Q_nominal_unit=W  Q_nominal_value=1
  Convection Roof to Internal : fl_lib/Thermal/Thermal Elements/Convective Heat Transfer  area=roof_area m^2  heat_tr_coeff=roof_heat_transfer_coeff_internal W/(m^2 * K)  T_specify=off  T_priority=None  T=0 K  T_nominal_specify=off  T_nominal_unit=K  T_nominal_value=1  Q_specify=off  Q_priority=None  Q=0 W  Q_nominal_specify=off  Q_nominal_unit=W  Q_nominal_value=1
  Convection Wall to External : fl_lib/Thermal/Thermal Elements/Convective Heat Transfer  area=wall_area m^2  heat_tr_coeff=wall_heat_transfer_coeff_external W/(m^2 * K)  T_specify=off  T_priority=None  T=0 K  T_nominal_specify=off  T_nominal_unit=K  T_nominal_value=1  Q_specify=off  Q_priority=None  Q=0 W  Q_nominal_specify=off  Q_nominal_unit=W  Q_nominal_value=1
  Convection Wall to Internal : fl_lib/Thermal/Thermal Elements/Convective Heat Transfer  area=wall_area m^2  heat_tr_coeff=wall_heat_transfer_coeff_internal W/(m^2 * K)  T_specify=off  T_priority=None  T=0 K  T_nominal_specify=off  T_nominal_unit=K  T_nominal_value=1  Q_specify=off  Q_priority=None  Q=0 W  Q_nominal_specify=off  Q_nominal_unit=W  Q_nominal_value=1
  External Temperature : fl_lib/Thermal/Thermal Sources/Controlled Temperature Source
  Floor Conduction : fl_lib/Thermal/Thermal Elements/Conductive Heat Transfer  area=floor_area m^2  thickness=floor_thickness m  th_cond=floor_conductivity W/(m*K)  T_specify=off  T_priority=None  T=0 K  T_nominal_specify=off  T_nominal_unit=K  T_nominal_value=1  Q_specify=off  Q_priority=None  Q=0 W  Q_nominal_specify=off  Q_nominal_unit=W  Q_nominal_value=1
  Ground Temperature : fl_lib/Thermal/Thermal Sources/Temperature Source  temperature=ground_temperature degC
  PS-Simulink Converter : nesl_utility/PS-Simulink Converter  PhysicalDomain=network_engine_domain  SubClassName=ps_output  LeftPortType=input  RightPortType=output  PseudoPeriodic=off  Frequencies=[]  Unit=degC  AffineConversion=on
  Roof Conduction External Side : fl_lib/Thermal/Thermal Elements/Conductive Heat Transfer  area=roof_area m^2  thickness=roof_thickness / 2 m  th_cond=roof_conductivity W/(m*K)  T_specify=off  T_priority=None  T=0 K  T_nominal_specify=off  T_nominal_unit=K  T_nominal_value=1  Q_specify=off  Q_priority=None  Q=0 W  Q_nominal_specify=off  Q_nominal_unit=W  Q_nominal_value=1
  Roof Conduction Internal Side : fl_lib/Thermal/Thermal Elements/Conductive Heat Transfer  area=roof_area m^2  thickness=roof_thickness / 2 m  th_cond=roof_conductivity W/(m*K)  T_specify=off  T_priority=None  T=0 K  T_nominal_specify=off  T_nominal_unit=K  T_nominal_value=1  Q_specify=off  Q_priority=None  Q=0 W  Q_nominal_specify=off  Q_nominal_unit=W  Q_nominal_value=1
  Roof Thermal Mass : fl_lib/Thermal/Thermal Elements/Thermal Mass  mass=roof_area * roof_thickness * wall_density kg  sp_heat=roof_specific_heat J/kg/K  T_specify=on  T_priority=High  T=roof_initial_temperature degC  T_nominal_specify=off  T_nominal_unit=K  T_nominal_value=1  Q_specify=off  Q_priority=None  Q=0 W  Q_nominal_specify=off  Q_nominal_unit=W  Q_nominal_value=1
  Simulink-PS Converter : nesl_utility/Simulink-PS Converter  PhysicalDomain=network_engine_domain  SubClassName=ps_input  LeftPortType=input  RightPortType=output  PseudoPeriodic=off  Frequencies=[]  NoiseDistribution=none  NoiseParameters=[]  Unit=degC  AffineConversion=on  FilteringAndDerivatives=provide  SimscapeFilterOrder=1  InputFilterTimeConstant=0.001  UdotUserProvided=0
  Temperature Sensor : fl_lib/Thermal/Thermal Sensors/Temperature Sensor
  Thermal Reference : fl_lib/Thermal/Thermal Elements/Thermal Reference
  Thermal Reference1 : fl_lib/Thermal/Thermal Elements/Thermal Reference
  Wall Conduction External Side : fl_lib/Thermal/Thermal Elements/Conductive Heat Transfer  area=wall_area m^2  thickness=wall_thickness / 2 m  th_cond=wall_conductivity W/(m*K)  T_specify=off  T_priority=None  T=0 K  T_nominal_specify=off  T_nominal_unit=K  T_nominal_value=1  Q_specify=off  Q_priority=None  Q=0 W  Q_nominal_specify=off  Q_nominal_unit=W  Q_nominal_value=1
  Wall Conduction Internal Side : fl_lib/Thermal/Thermal Elements/Conductive Heat Transfer  area=wall_area m^2  thickness=wall_thickness / 2 m  th_cond=wall_conductivity W/(m*K)  T_specify=off  T_priority=None  T=0 K  T_nominal_specify=off  T_nominal_unit=K  T_nominal_value=1  Q_specify=off  Q_priority=None  Q=0 W  Q_nominal_specify=off  Q_nominal_unit=W  Q_nominal_value=1
  Wall Thermal Mass : fl_lib/Thermal/Thermal Elements/Thermal Mass  mass=wall_area * wall_thickness * wall_density kg  sp_heat=wall_specific_heat J/kg/K  T_specify=on  T_priority=High  T=wall_initial_temperature degC  T_nominal_specify=off  T_nominal_unit=K  T_nominal_value=1  Q_specify=off  Q_priority=None  Q=0 W  Q_nominal_specify=off  Q_nominal_unit=W  Q_nominal_value=1
  Int : PMIOPort  Side=Right
  tag scope: T1=global
  wires:
  Ext/1 -> Simulink-PS Converter/1
  PS-Simulink Converter/1 -> [T1]
  connections:
  External Temperature/RConn1 -- Simulink-PS Converter/RConn1
  Wall Conduction Internal Side/RConn1 -- Convection Wall to Internal/LConn1
  Convection Roof to Internal/RConn1 -- Convection Floor to Internal/RConn1 -- Temperature Sensor/LConn1 -- Convection Wall to Internal/RConn1 -- Int/RConn1
  External Temperature/LConn1 -- Convection Wall to External/LConn1 -- Convection Roof to External/LConn1
  Wall Conduction External Side/LConn1 -- Convection Wall to External/RConn1
  Wall Thermal Mass/LConn1 -- Wall Conduction Internal Side/LConn1 -- Wall Conduction External Side/RConn1
  Roof Thermal Mass/LConn1 -- Roof Conduction Internal Side/LConn1 -- Roof Conduction External Side/RConn1
  Roof Conduction External Side/LConn1 -- Convection Roof to External/RConn1
  Roof Conduction Internal Side/RConn1 -- Convection Roof to Internal/LConn1
  Floor Conduction/RConn1 -- Convection Floor to Internal/LConn1
  Floor Conduction/LConn1 -- Ground Temperature/LConn1
  Thermal Reference1/LConn1 -- Temperature Sensor/RConn1
  Temperature Sensor/RConn2 -- PS-Simulink Converter/LConn1
  Thermal Reference/LConn1 -- External Temperature/RConn2

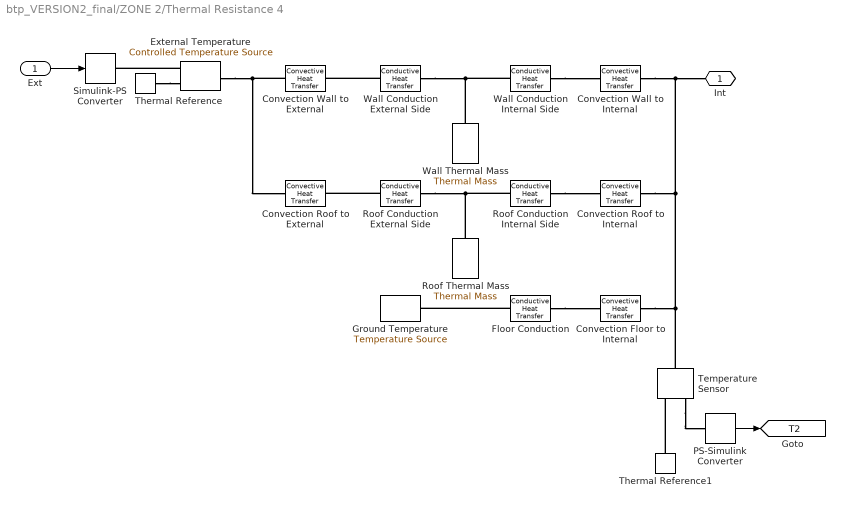
== system btp_VERSION2_final/ZONE 2/Thermal Resistance 4 ==
  Ext : Inport
  Convection Floor to Internal : fl_lib/Thermal/Thermal Elements/Convective Heat Transfer  area=floor_area m^2  heat_tr_coeff=floor_heat_transfer_coeff_internal W/(m^2 * K)  T_specify=off  T_priority=None  T=0 K  T_nominal_specify=off  T_nominal_unit=K  T_nominal_value=1  Q_specify=off  Q_priority=None  Q=0 W  Q_nominal_specify=off  Q_nominal_unit=W  Q_nominal_value=1
  Convection Roof to External : fl_lib/Thermal/Thermal Elements/Convective Heat Transfer  area=roof_area m^2  heat_tr_coeff=roof_heat_transfer_coeff_external W/(m^2 * K)  T_specify=off  T_priority=None  T=0 K  T_nominal_specify=off  T_nominal_unit=K  T_nominal_value=1  Q_specify=off  Q_priority=None  Q=0 W  Q_nominal_specify=off  Q_nominal_unit=W  Q_nominal_value=1
  Convection Roof to Internal : fl_lib/Thermal/Thermal Elements/Convective Heat Transfer  area=roof_area m^2  heat_tr_coeff=roof_heat_transfer_coeff_internal W/(m^2 * K)  T_specify=off  T_priority=None  T=0 K  T_nominal_specify=off  T_nominal_unit=K  T_nominal_value=1  Q_specify=off  Q_priority=None  Q=0 W  Q_nominal_specify=off  Q_nominal_unit=W  Q_nominal_value=1
  Convection Wall to External : fl_lib/Thermal/Thermal Elements/Convective Heat Transfer  area=wall_area m^2  heat_tr_coeff=wall_heat_transfer_coeff_external W/(m^2 * K)  T_specify=off  T_priority=None  T=0 K  T_nominal_specify=off  T_nominal_unit=K  T_nominal_value=1  Q_specify=off  Q_priority=None  Q=0 W  Q_nominal_specify=off  Q_nominal_unit=W  Q_nominal_value=1
  Convection Wall to Internal : fl_lib/Thermal/Thermal Elements/Convective Heat Transfer  area=wall_area m^2  heat_tr_coeff=wall_heat_transfer_coeff_internal W/(m^2 * K)  T_specify=off  T_priority=None  T=0 K  T_nominal_specify=off  T_nominal_unit=K  T_nominal_value=1  Q_specify=off  Q_priority=None  Q=0 W  Q_nominal_specify=off  Q_nominal_unit=W  Q_nominal_value=1
  External Temperature : fl_lib/Thermal/Thermal Sources/Controlled Temperature Source
  Floor Conduction : fl_lib/Thermal/Thermal Elements/Conductive Heat Transfer  area=floor_area m^2  thickness=floor_thickness m  th_cond=floor_conductivity W/(m*K)  T_specify=off  T_priority=None  T=0 K  T_nominal_specify=off  T_nominal_unit=K  T_nominal_value=1  Q_specify=off  Q_priority=None  Q=0 W  Q_nominal_specify=off  Q_nominal_unit=W  Q_nominal_value=1
  Ground Temperature : fl_lib/Thermal/Thermal Sources/Temperature Source  temperature=ground_temperature degC
  PS-Simulink Converter : nesl_utility/PS-Simulink Converter  PhysicalDomain=network_engine_domain  SubClassName=ps_output  LeftPortType=input  RightPortType=output  PseudoPeriodic=off  Frequencies=[]  Unit=degC  AffineConversion=on
  Roof Conduction External Side : fl_lib/Thermal/Thermal Elements/Conductive Heat Transfer  area=roof_area m^2  thickness=roof_thickness / 2 m  th_cond=roof_conductivity W/(m*K)  T_specify=off  T_priority=None  T=0 K  T_nominal_specify=off  T_nominal_unit=K  T_nominal_value=1  Q_specify=off  Q_priority=None  Q=0 W  Q_nominal_specify=off  Q_nominal_unit=W  Q_nominal_value=1
  Roof Conduction Internal Side : fl_lib/Thermal/Thermal Elements/Conductive Heat Transfer  area=roof_area m^2  thickness=roof_thickness / 2 m  th_cond=roof_conductivity W/(m*K)  T_specify=off  T_priority=None  T=0 K  T_nominal_specify=off  T_nominal_unit=K  T_nominal_value=1  Q_specify=off  Q_priority=None  Q=0 W  Q_nominal_specify=off  Q_nominal_unit=W  Q_nominal_value=1
  Roof Thermal Mass : fl_lib/Thermal/Thermal Elements/Thermal Mass  mass=roof_area * roof_thickness * wall_density kg  sp_heat=roof_specific_heat J/kg/K  T_specify=on  T_priority=High  T=roof_initial_temperature degC  T_nominal_specify=off  T_nominal_unit=K  T_nominal_value=1  Q_specify=off  Q_priority=None  Q=0 W  Q_nominal_specify=off  Q_nominal_unit=W  Q_nominal_value=1
  Simulink-PS Converter : nesl_utility/Simulink-PS Converter  PhysicalDomain=network_engine_domain  SubClassName=ps_input  LeftPortType=input  RightPortType=output  PseudoPeriodic=off  Frequencies=[]  NoiseDistribution=none  NoiseParameters=[]  Unit=degC  AffineConversion=on  FilteringAndDerivatives=provide  SimscapeFilterOrder=1  InputFilterTimeConstant=0.001  UdotUserProvided=0
  Temperature Sensor : fl_lib/Thermal/Thermal Sensors/Temperature Sensor
  Thermal Reference : fl_lib/Thermal/Thermal Elements/Thermal Reference
  Thermal Reference1 : fl_lib/Thermal/Thermal Elements/Thermal Reference
  Wall Conduction External Side : fl_lib/Thermal/Thermal Elements/Conductive Heat Transfer  area=wall_area m^2  thickness=wall_thickness / 2 m  th_cond=wall_conductivity W/(m*K)  T_specify=off  T_priority=None  T=0 K  T_nominal_specify=off  T_nominal_unit=K  T_nominal_value=1  Q_specify=off  Q_priority=None  Q=0 W  Q_nominal_specify=off  Q_nominal_unit=W  Q_nominal_value=1
  Wall Conduction Internal Side : fl_lib/Thermal/Thermal Elements/Conductive Heat Transfer  area=wall_area m^2  thickness=wall_thickness / 2 m  th_cond=wall_conductivity W/(m*K)  T_specify=off  T_priority=None  T=0 K  T_nominal_specify=off  T_nominal_unit=K  T_nominal_value=1  Q_specify=off  Q_priority=None  Q=0 W  Q_nominal_specify=off  Q_nominal_unit=W  Q_nominal_value=1
  Wall Thermal Mass : fl_lib/Thermal/Thermal Elements/Thermal Mass  mass=wall_area * wall_thickness * wall_density kg  sp_heat=wall_specific_heat J/kg/K  T_specify=on  T_priority=High  T=wall_initial_temperature degC  T_nominal_specify=off  T_nominal_unit=K  T_nominal_value=1  Q_specify=off  Q_priority=None  Q=0 W  Q_nominal_specify=off  Q_nominal_unit=W  Q_nominal_value=1
  Int : PMIOPort  Side=Right
  tag scope: T2=global
  wires:
  PS-Simulink Converter/1 -> [T2]
  Ext/1 -> Simulink-PS Converter/1
  connections:
  Thermal Reference/LConn1 -- External Temperature/RConn2
  Temperature Sensor/RConn2 -- PS-Simulink Converter/LConn1
  Thermal Reference1/LConn1 -- Temperature Sensor/RConn1
  Floor Conduction/LConn1 -- Ground Temperature/LConn1
  Floor Conduction/RConn1 -- Convection Floor to Internal/LConn1
  Roof Conduction Internal Side/RConn1 -- Convection Roof to Internal/LConn1
  Roof Conduction External Side/LConn1 -- Convection Roof to External/RConn1
  Roof Conduction Internal Side/LConn1 -- Roof Thermal Mass/LConn1 -- Roof Conduction External Side/RConn1
  Wall Conduction Internal Side/LConn1 -- Wall Thermal Mass/LConn1 -- Wall Conduction External Side/RConn1
  Wall Conduction External Side/LConn1 -- Convection Wall to External/RConn1
  Convection Wall to External/LConn1 -- Convection Roof to External/LConn1 -- External Temperature/LConn1
  Convection Floor to Internal/RConn1 -- Int/RConn1 -- Convection Wall to Internal/RConn1 -- Convection Roof to Internal/RConn1 -- Temperature Sensor/LConn1
  Wall Conduction Internal Side/RConn1 -- Convection Wall to Internal/LConn1
  External Temperature/RConn1 -- Simulink-PS Converter/RConn1

== matlab function btp_VERSION2_final/Ventilation Unit/MATLAB Function1 ==
  data: u input; y output
function y = fcn(u)
if u>0.9
    y=1;
else
    y=0;
end
end

== matlab function btp_VERSION2_final/Ventilation Unit/MATLAB Function ==
  data: u input; y output
function y = fcn(u)
if u>0.9
    y=1.002;
else
    y=0.098;
end

== matlab function btp_VERSION2_final/Ventilation Unit/Machine learning model/MATLAB Function2 ==
  data: y output size=5; X input; Y1 input
function y = fcn(X,Y1)
coder.extrinsic('regress')
coder.extrinsic('print')
%x1 = evalin('base','dbresponses22S1');
%X = zeros(500,5);
%X = [x1(1,:) x1(2,:) x1(5,:) x1(6,:) x1(7,:)];
%Y = zeros(500,1);
%Y1 = x1(4,:);
%b = zeros(5);
y= zeros(5,1);
y = regress(Y1,X);

== matlab function btp_VERSION2_final/Ventilation Unit/Machine learning model/MATLAB Function3 ==
  data: u input size=5; y output; data input
function y = fcn(u, data)
y = u(1)*20+ u(2)*1+ u(3)*179+ u(4)*70+ u(5)*data;
